simulink model "Toyota_CHR_Climate_Model_V2"  (R2025a)
settings: Solver=ode15s  StartTime=0.0  StopTime=100  MaxStep=0.01  RelTol=1e-3
libraries: slpidlib x1
settings Model: Creator=user  LastModifiedBy=user

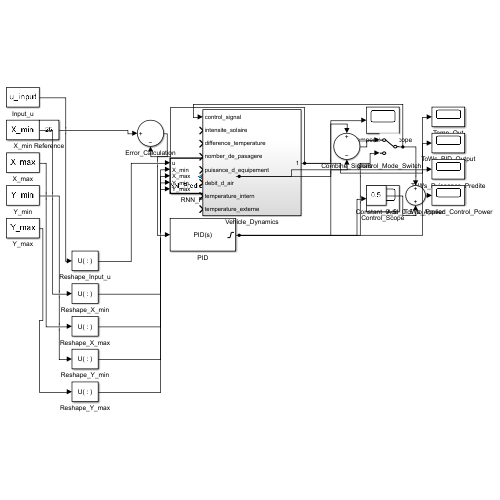
[thumbnail: Simulink's stored preview of the top-level diagram]
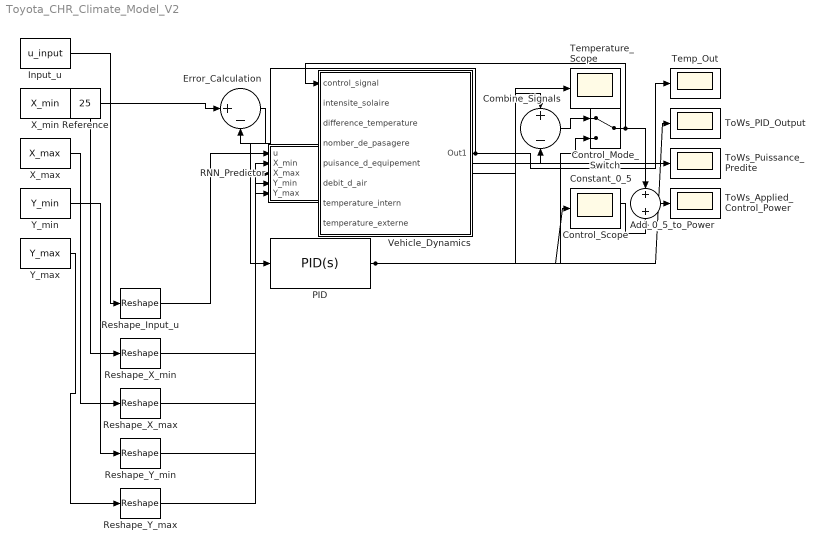
== system Toyota_CHR_Climate_Model_V2 ==
  Add_0_5_to_Power : Sum
  Combine_Signals : Sum  Inputs=+-
  Constant_0_5 : Constant  Value=0.5
  Control_Mode_Switch : ManualSwitch
  Control_Scope : Scope
  Error_Calculation : Sum  Inputs=|+-
  Input_u : FromWorkspace  VariableName=u_input
  PID : slpidlib/PID Controller  Controller=PID  Form=Parallel  TimeDomain=Continuous-time  UseExternalTs=off  SampleTime=-1  IntegratorMethod=Forward Euler  FilterMethod=Forward Euler  ControllerParametersSource=internal  P=0.5  I=0.05  UseKiTs=off  D=0  UseExternalDerivativeSource=off  N=100  UseFilter=on  TunerSelectOption=Transfer Function Based (PID Tuner App)  InitialConditionSource=internal  InitialConditionForIntegrator=0  InitialConditionForFilter=0  DifferentiatorICPrevScaledInput=0  ExternalReset=none  TrackingMode=off  Kt=1  LimitOutput=on  SatLimitsSource=internal  UpperSaturationLimit=1  LowerSaturationLimit=-1  LinearizeAsGain=on  AntiWindupMode=none  Kb=1  LimitIntegrator=off  UpperIntegratorSaturationLimit=inf  LowerIntegratorSaturationLimit=-inf  POutMin=[]  POutMax=[]  IOutMin=[]  IOutMax=[]  DOutMin=[]  DOutMax=[]  NOutMin=[]  NOutMax=[]  SumOutMin=[]  SumOutMax=[]  SaturationOutMin=[]  SaturationOutMax=[]  PParamMin=[]  PParamMax=[]  IParamMin=[]  IParamMax=[]  DParamMin=[]  DParamMax=[]  NParamMin=[]  NParamMax=[]  KbParamMin=[]  KbParamMax=[]  KtParamMin=[]  KtParamMax=[]  KbOutMin=[]  KbOutMax=[]  KtOutMin=[]  KtOutMax=[]  IntegratorOutMin=[]  IntegratorOutMax=[]  FilterOutMin=[]  FilterOutMax=[]  SumI1OutMin=[]  SumI1OutMax=[]  SumI2OutMin=[]  SumI2OutMax=[]  SumI3OutMin=[]  SumI3OutMax=[]  SumI4OutMin=[]  SumI4OutMax=[]  SumDOutMin=[]  SumDOutMax=[]  DifferentiatorOutMin=[]  DifferentiatorOutMax=[]  FilterDiffOutCoefMin=[]  FilterDiffOutCoefMax=[]  ReciprocalOutMin=[]  ReciprocalOutMax=[]  SumDenOutMin=[]  SumDenOutMax=[]  SumNumOutMin=[]  SumNumOutMax=[]  DivideOutMin=[]  DivideOutMax=[]  UdiffTsProdOutMin=[]  UdiffTsProdOutMax=[]  NTsProdOutMin=[]  NTsProdOutMax=[]  UintegralTsProdOutMin=[]  UintegralTsProdOutMax=[]  UngainTsProdOutMin=[]  UngainTsProdOutMax=[]  ClampingZeroOutDataTypeStr=Inherit: Inherit via back propagation  ClampingZeroOutMin=[]  ClampingZeroOutMax=[]  FilterDenConstantOutDataTypeStr=Inherit: Inherit via back propagation  FilterDenConstantOutMin=[]  FilterDenConstantOutMax=[]  PCopyOutDataTypeStr=Inherit: Inherit via back propagation  PCopyOutMin=[]  PCopyOutMax=[]  NCopyOutDataTypeStr=Inherit: Inherit via back propagation  NCopyOutMin=[]  NCopyOutMax=[]  IntegratorContinuousStateAttributes=''  IntegratorStateMustResolveToSignalObject=off  IntegratorRTWStateStorageClass=Auto  FilterContinuousStateAttributes=''  FilterStateMustResolveToSignalObject=off  FilterRTWStateStorageClass=Auto  ParallelPVariant=InternalParameters  IdealPVariant=Disabled  IVariant=InternalParameters  DVariant=InternalParameters  IntegratorVariant=Continuous  SatVariant=Enabled  AWVariant=Passthrough  PCopyVariant=Disabled  TRVariant=Disabled  FdbkBlocksVariant=Forward  IdealPFdbkVariant=Disabled  SatFdbkVariant=Disabled  DerivativeFilterVariant=ContFilter  NVariant=InternalParameters  NCopyVariant=Disabled  FilterICVariant=InternalICsFilter  IntegratorICVariant=InternalICs  ExternalResetVariant=Disabled  TRSumVariant=Passthrough  SumFdbkVariant=Disabled  SumVariant=Sum_PID  TsampFilterVariant=InternalTs  TsampNgainVariant=Passthrough  TsampIntegralVariant=Disabled_SignalSpec  ExternalSaturationOutDataTypeStr=Inherit: Same as second input  DerivativeSourceVariant=ErrorSignal  PreIntVariant=InternalPreInt
  RNN_Predictor : MATLAB Function  TreatAsAtomicUnit=on
  Reference : Constant  Value=25
  Reshape_Input_u : Reshape
  Reshape_X_max : Reshape
  Reshape_X_min : Reshape
  Reshape_Y_max : Reshape
  Reshape_Y_min : Reshape
  Temp_Out : Scope
  Temperature_Scope : Scope
  ToWs_Applied_Control_Power : Scope
  ToWs_PID_Output : Scope
  ToWs_Puissance_Predite : Scope
  Vehicle_Dynamics : Subsystem
  X_max : FromWorkspace  VariableName=X_max
  X_min : FromWorkspace  VariableName=X_min
  Y_max : FromWorkspace  VariableName=Y_max
  Y_min : FromWorkspace  VariableName=Y_min
  wires:
  Input_u/1 -> Reshape_Input_u/1
  X_min/1 -> Reshape_X_min/1
  X_max/1 -> Reshape_X_max/1
  Y_min/1 -> Reshape_Y_min/1
  Y_max/1 -> Reshape_Y_max/1
  Reshape_Input_u/1 -> RNN_Predictor/1(u)
  Reshape_X_min/1 -> RNN_Predictor/2(X_min)
  Reshape_X_max/1 -> RNN_Predictor/3(X_max)
  Reshape_Y_min/1 -> RNN_Predictor/4(Y_min)
  Reshape_Y_max/1 -> RNN_Predictor/5(Y_max)
  Error_Calculation/1 -> PID/1
  PID/1 -> Combine_Signals/1, Control_Mode_Switch/2, Control_Scope/1, ToWs_PID_Output/1
  RNN_Predictor/1(y) -> Combine_Signals/2, ToWs_Puissance_Predite/1
  Combine_Signals/1 -> Control_Mode_Switch/1
  Control_Mode_Switch/1 -> Vehicle_Dynamics/1(control_signal), Add_0_5_to_Power/1
  Reference/1 -> Error_Calculation/1
  Vehicle_Dynamics/1(Out1) -> Error_Calculation/2, Temperature_Scope/1, Temp_Out/1
  Constant_0_5/1 -> Add_0_5_to_Power/2
  Add_0_5_to_Power/1 -> ToWs_Applied_Control_Power/1

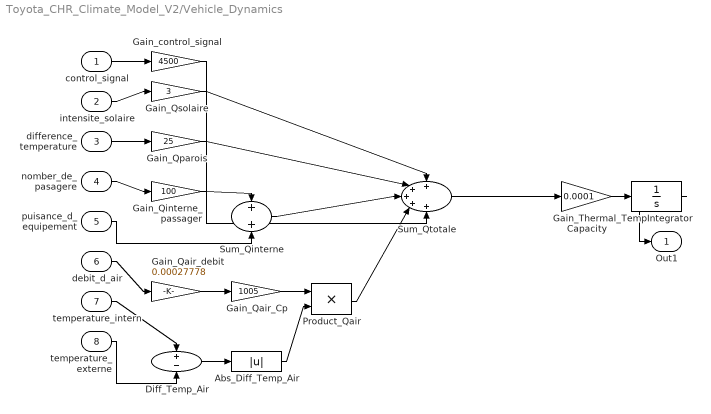
== system Toyota_CHR_Climate_Model_V2/Vehicle_Dynamics ==
  control_signal : Inport
  intensite_solaire : Inport  Port=2
  difference_temperature : Inport  Port=3
  nomber_de_pasagere : Inport  Port=4
  puisance_d_equipement : Inport  Port=5
  debit_d_air : Inport  Port=6
  temperature_intern : Inport  Port=7
  temperature_externe : Inport  Port=8
  Abs_Diff_Temp_Air : Abs  SaturateOnIntegerOverflow=off
  Diff_Temp_Air : Sum  Inputs=+-
  Gain_Qair_Cp : Gain  Gain=1005
  Gain_Qair_debit : Gain  Gain=0.00027778
  Gain_Qinterne_passager : Gain  Gain=100
  Gain_Qparois : Gain  Gain=25
  Gain_Qsolaire : Gain  Gain=3
  Gain_Thermal_Capacity : Gain  Gain=0.0001
  Gain_control_signal : Gain  Gain=4500
  Product_Qair : Product
  Sum_Qinterne : Sum
  Sum_Qtotale : Sum  Inputs=+++++
  TempIntegrator : Integrator  InitialCondition=20
  Out1 : Outport
  wires:
  ? -> ?
  intensite_solaire/1 -> Gain_Qsolaire/1
  difference_temperature/1 -> Gain_Qparois/1
  nomber_de_pasagere/1 -> Gain_Qinterne_passager/1
  Gain_Qinterne_passager/1 -> Sum_Qinterne/1
  puisance_d_equipement/1 -> Sum_Qinterne/2
  debit_d_air/1 -> Gain_Qair_debit/1
  Gain_Qair_debit/1 -> Gain_Qair_Cp/1
  temperature_intern/1 -> Diff_Temp_Air/1
  temperature_externe/1 -> Diff_Temp_Air/2
  Diff_Temp_Air/1 -> Abs_Diff_Temp_Air/1
  Gain_Qair_Cp/1 -> Product_Qair/1
  Abs_Diff_Temp_Air/1 -> Product_Qair/2
  control_signal/1 -> Gain_control_signal/1
  Gain_Qsolaire/1 -> Sum_Qtotale/1
  Gain_Qparois/1 -> Sum_Qtotale/2
  Sum_Qinterne/1 -> Sum_Qtotale/3
  Product_Qair/1 -> Sum_Qtotale/4
  Gain_control_signal/1 -> Sum_Qtotale/5
  Sum_Qtotale/1 -> Gain_Thermal_Capacity/1
  Gain_Thermal_Capacity/1 -> TempIntegrator/1
  TempIntegrator/1 -> Out1/1

== matlab function Toyota_CHR_Climate_Model_V2/RNN_Predictor ==
  data: u input; y output; X_min input; X_max input; Y_min input; Y_max input
function y = RNN_Predictor_Function(u, X_min, X_max, Y_min, Y_max)
%#codegen

%% Initializations for code generation
y = 0; % Initialize output

%% Protection against division by zero
epsilon = 1e-6;
range_x = X_max(:) - X_min(:);
range_x(abs(range_x) < epsilon) = epsilon;

%% Input Normalization (mapminmax from training)
x_norm = (u(:) - X_min(:)) ./ range_x;

%% Persistent delay states for RNN
persistent ai1 ai2
if isempty(ai1)
    ai1 = zeros(20, 2); % Layer 1 delay states
end
if isempty(ai2)
    ai2 = zeros(10, 2); % Layer 2 delay states
end

%% Call RNN prediction function
[y_norm, ai1, ai2] = predictRNN(x_norm, ai1, ai2);

%% Denormalize output
y = double(y_norm) * (Y_max - Y_min) + Y_min;

% Clamp output to a physically reasonable range to prevent runaway values
% Adjust the range as needed for your system
y = max(min(y, 1), -1);

end
